simulink model "Resp18e_updatedPulse"  (Simulink 7.3)
settings: Solver=ode23  StartTime=0.0  StopTime=20  FixedStep=0.01  MaxStep=0.05  RelTol=1e-6
values from neighbouring files (symbols this model uses):
  alpha_CO2_brain = 2.9/1e3*760/P_stp/K_stp    (= 0.00097047576489)    [initialize_parameters.m]
  alpha_CO2_fat = 0.9/K_stp/P_stp    (= 0.000396292281489)    [initialize_parameters.m]
  alpha_CO2_heart = 2.4/1e3*760/P_stp/K_stp    (= 0.00080315235715)    [initialize_parameters.m]
  alpha_CO2_lean = 4.2/1e3*760/P_stp/K_stp    (= 0.00140551662501)    [initialize_parameters.m]
  alpha_CO2_lungtiss_fast = alpha_CO2_lungtiss_fast./0.1333    [initialize_parameters.m]
  alpha_CO2_muscle = 4.2/1e3*760/P_stp/K_stp    (= 0.00140551662501)    [initialize_parameters.m]
  alpha_CO2_other = 3.0/1e3*760/P_stp/K_stp    (= 0.00100394044644)    [initialize_parameters.m]
  alpha_O2_fat = 5*0.024/K_stp/P_stp    (= 5.28389708651e-05)    [initialize_parameters.m]
  alpha_O2_tissue = 0.024/K_stp/P_stp    (= 1.0567794173e-05)    [initialize_parameters.m]
  BOHRF0 = O2_SHIFT - T_BLOOD_M_37 * (0.024 + BOHRF * 0.0147) - BOHRF1 * 7.4    (= -3.552)    [initialize_parameters.m]
  BOHRF1 = BOHRF * (1 - T_BLOOD_M_37 * 0.0065)    (= 0.48)    [initialize_parameters.m]
  C_a_CO2_i = 20.8e-3    (= 0.0208)    [initialize_parameters.m]    (also in resp18e_ic_norm.mat = 0.0202734801806)
  C_a_O2_i = 8.95e-3    (= 0.00895)    [initialize_parameters.m]    (also in resp18e_ic_norm.mat = 0.00918087581167)
  CAP_O2 = 0.01 * CAP_O2    (= 0.201)    [initialize_parameters.m]
  Cardiac_duty_cycle = 40    [initialize_parameters.m]
  Co_CO2_brain = 401*K_Co_CO2/1e3/K_stp    (= 0.0107345869894)    [initialize_parameters.m]
  Co_CO2_heart = 487*K_Co_CO2/1e3/K_stp    (= 0.0130367677403)    [initialize_parameters.m]
  Co_CO2_lean = 342*K_Co_CO2/1e3/K_stp    (= 0.00915518391618)    [initialize_parameters.m]
  Co_CO2_muscle = 342*K_Co_CO2/1e3/K_stp    (= 0.00915518391618)    [initialize_parameters.m]
  Co_CO2_other = 355*K_Co_CO2/1e3/K_stp    (= 0.00950318798317)    [initialize_parameters.m]
  DH2ODS = DH2ODS + 0.007 * HB_MEQ * (HB_MEQ - 9) / (13.5 * (13.5 - 9))    (= 0.00498709726946)    [initialize_parameters.m]
  F_insp_alv_alvds = F_v_alv_deadspace / F_insp_hivq    (= 0.00299401197605)    [initialize_parameters.m]
  F_insp_alv_hivq = F_v_alv_hivq      / F_insp_hivq    (= 0.997005988024)    [initialize_parameters.m]
  F_insp_alv_lovq = F_v_alv_lovq      / F_insp_lovq    (= 0.5)    [initialize_parameters.m]
  F_insp_alv_midvq = F_v_alv_midvq     / F_insp_lovq    (= 0.5)    [initialize_parameters.m]
  F_insp_hivq = F_v_alv_deadspace + F_v_alv_hivq    (= 0.334)    [initialize_parameters.m]
  F_insp_lovq = F_v_alv_midvq     + F_v_alv_lovq    (= 0.666)    [initialize_parameters.m]
  Fi_CO2_param_est = 0.01    [initialize_parameters.m]
  Fi_error = 1e-6    (= 1e-06)    [initialize_parameters.m]
  Fi_N2_mean = 1-(Fi_O2_mean + Fi_N2O_mean)    (= 0.65)    [initialize_parameters.m]
  Fi_O2_mean = 0.35    [initialize_parameters.m]
  Fi_O2_param_est = 0.01    [initialize_parameters.m]
  Fq_brain = 0.114    [initialize_parameters.m]
  Fq_error = 1e-8    (= 1e-08)    [initialize_parameters.m]
  Fq_fat = 0.103    [initialize_parameters.m]
  Fq_heart = 0.041    [initialize_parameters.m]
  Fq_hepatic = 0.069    [initialize_parameters.m]
  Fq_kidneys = 0.215    [initialize_parameters.m]
  Fq_lean = 0.090    (= 0.09)    [initialize_parameters.m]
  Fq_lungs_anatomicalshunt = 0.01    [initialize_parameters.m]
  Fq_lungs_hivq = (1-Fq_lungs_pulmshunt-Fq_lungs_anatomicalshunt)    *F_v_alv_hivq/(F_v_alv_hivq+F_v_alv_midvq+F_v_alv_lovq)    (= 0.3)    [initialize_parameters.m]
  Fq_lungs_lovq = (1-Fq_lungs_pulmshunt-Fq_lungs_anatomicalshunt)    *F_v_alv_lovq/(F_v_alv_hivq+F_v_alv_midvq+F_v_alv_lovq)    (= 0.3)    [initialize_parameters.m]
  Fq_lungs_midvq = (1-Fq_lungs_pulmshunt-Fq_lungs_anatomicalshunt)    *F_v_alv_midvq/(F_v_alv_hivq+F_v_alv_midvq+F_v_alv_lovq)    (= 0.3)    [initialize_parameters.m]
  Fq_lungs_pulmshunt = 0.09    [initialize_parameters.m]
  Fq_muscle = 0.096    [initialize_parameters.m]
  Fq_pershunt = 0.101    [initialize_parameters.m]
  Fq_portal = 0.171    [initialize_parameters.m]
  FRC = 2.2    [initialize_parameters.m]
  H2OB = H2OVC + 0.938 * (1 - VC_74)    (= 0.840191964286)    [initialize_parameters.m]
  k_CO2_lungtiss_fast_alvds = k_CO2_lungtiss_fast*F_v_alv_deadspace    (= 3.63090772693e-07)    [initialize_parameters.m]
  k_CO2_lungtiss_fast_hivq = k_CO2_lungtiss_fast*F_v_alv_hivq    (= 0.000120909227307)    [initialize_parameters.m]
  k_CO2_lungtiss_fast_lovq = k_CO2_lungtiss_fast*F_v_alv_lovq    (= 0.000120909227307)    [initialize_parameters.m]
  k_CO2_lungtiss_fast_midvq = k_CO2_lungtiss_fast*F_v_alv_midvq    (= 0.000120909227307)    [initialize_parameters.m]
  k_CO2_lungtiss_slow_alvds = k_CO2_lungtiss_slow*F_v_alv_deadspace    (= 4.95123780945e-09)    [initialize_parameters.m]
  k_CO2_lungtiss_slow_hivq = k_CO2_lungtiss_slow*F_v_alv_hivq    (= 1.64876219055e-06)    [initialize_parameters.m]
  k_CO2_lungtiss_slow_lovq = k_CO2_lungtiss_slow*F_v_alv_lovq    (= 1.64876219055e-06)    [initialize_parameters.m]
  k_CO2_lungtiss_slow_midvq = k_CO2_lungtiss_slow*F_v_alv_midvq    (= 1.64876219055e-06)    [initialize_parameters.m]
  K_diff_CO2_hivq = K_diff_CO2*F_v_alv_hivq    (= 0.0014985)    [initialize_parameters.m]
  K_diff_CO2_lovq = K_diff_CO2*F_v_alv_lovq    (= 0.0014985)    [initialize_parameters.m]
  K_diff_CO2_midvq = K_diff_CO2*F_v_alv_midvq    (= 0.0014985)    [initialize_parameters.m]
  K_diff_O2_hivq = K_diff_O2*F_v_alv_hivq    (= 7.326e-05)    [initialize_parameters.m]
  K_diff_O2_lovq = K_diff_O2*F_v_alv_lovq    (= 7.326e-05)    [initialize_parameters.m]
  K_diff_O2_midvq = K_diff_O2*F_v_alv_midvq    (= 7.326e-05)    [initialize_parameters.m]
  K_exp_alv_alvds = 1/1    (= 1)    [initialize_parameters.m]
  K_exp_alv_hivq = 1/1    (= 1)    [initialize_parameters.m]
  K_press = 760/101.325    (= 7.50061682704)    [initialize_parameters.m]
  K_stp = R*(T_stp+273.15)/(P_stp*1000)    (= 22.4135311621)    [initialize_parameters.m]
  Kg_alv = R*(T_alv+273.15)/(P_baro*1000)    (= 25.3668469802)    [initialize_parameters.m]
  LN10 = 2.30258509299405    (= 2.30258509299)    [initialize_parameters.m]
  m_alv_alvds_i = (FRC-V_deadspace_total)/Kg_alv * F_v_alv_deadspace    [initialize_parameters.m]
  m_alv_hivq_i = (FRC-V_deadspace_total)/Kg_alv * F_v_alv_hivq    [initialize_parameters.m]
  m_alv_lovq_i = (FRC-V_deadspace_total)/Kg_alv * F_v_alv_lovq    [initialize_parameters.m]
  m_alv_midvq_i = (FRC-V_deadspace_total)/Kg_alv * F_v_alv_midvq    [initialize_parameters.m]
  m_CO2_alv_alvds_i = F_CO2_i * m_alv_alvds_i    [initialize_parameters.m]
  m_CO2_alv_hivq_i = F_CO2_i * m_alv_hivq_i    [initialize_parameters.m]
  m_CO2_alv_lovq_i = F_CO2_i * m_alv_lovq_i    [initialize_parameters.m]
  m_CO2_alv_midvq_i = F_CO2_i * m_alv_midvq_i    [initialize_parameters.m]
  m_CO2_brain_b_i = C_a_CO2_i*Vb_brain    (= 0.002184)    [initialize_parameters.m]
  m_CO2_brain_t_i = (Co_CO2_brain  + alpha_CO2_brain *P_v_CO2_i)* Vt_brain    (= 0.0171268217946)    [initialize_parameters.m]
  m_CO2_common_b_i = C_a_CO2_i*Vb_common    (= 0.0170421333333)    [initialize_parameters.m]
  m_CO2_ds0_i = F_CO2_i*m_ds0_i    (= 0.000985538329597)    [initialize_parameters.m]
  m_CO2_ds_large_i = F_CO2_i * m_deadspace_large_1    [initialize_parameters.m]
  m_CO2_ds_med_hivq1_i = F_CO2_i * m_deadspace_med_hivq_1    [initialize_parameters.m]
  m_CO2_ds_med_hivq2_i = F_CO2_i * m_deadspace_med_hivq_2    [initialize_parameters.m]
  m_CO2_ds_med_lovq1_i = F_CO2_i * m_deadspace_med_lovq_1    [initialize_parameters.m]
  m_CO2_ds_med_lovq2_i = F_CO2_i * m_deadspace_med_lovq_2    [initialize_parameters.m]
  m_CO2_ds_small_alvds_i = F_CO2_i * m_deadspace_small_alvdeadspace    [initialize_parameters.m]
  m_CO2_ds_small_hivq_i = F_CO2_i * m_deadspace_small_hivq    [initialize_parameters.m]
  m_CO2_ds_small_lovq_i = F_CO2_i * m_deadspace_small_lovq    [initialize_parameters.m]
  m_CO2_ds_small_midvq_i = F_CO2_i * m_deadspace_small_midvq    [initialize_parameters.m]
  m_CO2_fat_b_i = C_a_CO2_i*Vb_fat    (= 0.0116896)    [initialize_parameters.m]
  m_CO2_fat_t_i = P_a_CO2_i*alpha_CO2_fat*Vt_fat    (= 0.0302752719501)    [initialize_parameters.m]
  m_CO2_heart_b_i = C_a_CO2_i*Vb_heart    (= 0.000832)    [initialize_parameters.m]
  m_CO2_heart_t_i = (Co_CO2_heart  + alpha_CO2_heart *P_v_CO2_i)* Vt_heart    (= 0.00402544335149)    [initialize_parameters.m]
  m_CO2_hepatic_b_i = C_a_CO2_i*Vb_hepatic    (= 0.0019136)    [initialize_parameters.m]
  m_CO2_kidneys_b_i = C_a_CO2_i*Vb_kidneys    (= 0.0012064)    [initialize_parameters.m]
  m_CO2_kidneys_t_i = (Co_CO2_other  + alpha_CO2_other *P_v_CO2_i)* Vt_kidneys    (= 0.0045902552907)    [initialize_parameters.m]
  m_CO2_lean_b_i = C_a_CO2_i*Vb_lean    (= 0.0191984)    [initialize_parameters.m]
  m_CO2_lean_t_i = (Co_CO2_lean   + alpha_CO2_lean  *P_v_CO2_i)* Vt_lean    (= 0.0884995401953)    [initialize_parameters.m]
  m_CO2_liver_t_i = (Co_CO2_other  + alpha_CO2_other *P_v_CO2_i)* Vt_liver    (= 0.0187019339777)    [initialize_parameters.m]
  m_CO2_lungtiss_fast_alvds_i = F_CO2_i*(P_baro-P_A_H2O)*V_lungtiss_alvds *alpha_CO2_lungtiss_fast(2)    [initialize_parameters.m]
  m_CO2_lungtiss_fast_hivq_i = F_CO2_i*(P_baro-P_A_H2O)*V_lungtiss_hivq  *alpha_CO2_lungtiss_fast(2)    [initialize_parameters.m]
  m_CO2_lungtiss_fast_lovq_i = F_CO2_i*(P_baro-P_A_H2O)*V_lungtiss_lovq  *alpha_CO2_lungtiss_fast(2)    [initialize_parameters.m]
  m_CO2_lungtiss_fast_midvq_i = F_CO2_i*(P_baro-P_A_H2O)*V_lungtiss_midvq *alpha_CO2_lungtiss_fast(2)    [initialize_parameters.m]
  m_CO2_lungtiss_slow_alvds_i = F_CO2_i*(P_baro-P_A_H2O)*V_lungtiss_alvds*alpha_CO2_lungtiss_slow    [initialize_parameters.m]
  m_CO2_lungtiss_slow_hivq_i = F_CO2_i*(P_baro-P_A_H2O)*V_lungtiss_hivq *alpha_CO2_lungtiss_slow    [initialize_parameters.m]
  m_CO2_lungtiss_slow_lovq_i = F_CO2_i*(P_baro-P_A_H2O)*V_lungtiss_lovq *alpha_CO2_lungtiss_slow    [initialize_parameters.m]
  m_CO2_lungtiss_slow_midvq_i = F_CO2_i*(P_baro-P_A_H2O)*V_lungtiss_midvq*alpha_CO2_lungtiss_slow    [initialize_parameters.m]
  m_CO2_LV_b_i = C_a_CO2_i*Vb_LV    (= 0.00391733333333)    [initialize_parameters.m]
  m_CO2_muscle_b_i = C_a_CO2_i*Vb_muscle    (= 0.0201344)    [initialize_parameters.m]
  m_CO2_muscle_t_i = (Co_CO2_muscle + alpha_CO2_muscle*P_v_CO2_i)* Vt_muscle    (= 0.363660431061)    [initialize_parameters.m]
  m_CO2_pershunt_b_i = C_a_CO2_i*Vb_pershunt    (= 0.0027248)    [initialize_parameters.m]
  m_CO2_portal_b_i = C_a_CO2_i*Vb_portal    (= 0.0210912)    [initialize_parameters.m]
  m_CO2_portal_t_i = (Co_CO2_other  + alpha_CO2_other *P_v_CO2_i)* Vt_portal    (= 0.0164739329706)    [initialize_parameters.m]
  m_CO2_pulmcap_b_hivq_i = C_a_CO2_i*Vb_pulmcap_hivq    (= 0.000630933333333)    [initialize_parameters.m]
  m_CO2_pulmcap_b_lovq_i = C_a_CO2_i*Vb_pulmcap_lovq    (= 0.000630933333333)    [initialize_parameters.m]
  m_CO2_pulmcap_b_midvq_i = C_a_CO2_i*Vb_pulmcap_midvq    (= 0.000630933333333)    [initialize_parameters.m]
  m_CO2_pulmcap_b_pulmshunt_i = C_a_CO2_i*Vb_pulmcap_pulmshunt    (= 0.0001872)    [initialize_parameters.m]
  m_CO2_RV_b_i = C_v_CO2_i*Vb_RV    (= 0.004181)    [initialize_parameters.m]
  m_N2_alv_alvds_i = Fi_N2_mean * (m_alv_alvds_i - m_CO2_alv_alvds_i)    [initialize_parameters.m]
  ... (+122 more)
undefined symbols (not defined in the file or in its folder): AH2OVC, AHCO3B, DHCO3BDS, litres, mole
libraries: simulink x28
(part 7 of 8)

== system Resp18e_updatedPulse/Patient/Kidneys/Kidneys/Blood gas curves Olszowka SI Units ==
  P_CO2 : Inport  OutDataType=sfix(16)  OutScaling=2^0
  P_O2 : Inport  Port=2  OutDataType=sfix(16)  OutScaling=2^0
  Olszowka's diss curves : Subsystem
  kPa > mm Hg : Gain  Gain=K_press  ParameterDataType=sfix(16)  ParameterScaling=2^0  OutDataType=sfix(16)  OutScaling=2^0  SaturateOnIntegerOverflow=on  OutDataTypeStr=Inherit: Same as input  ParamDataTypeStr=Inherit: Same as input
  kPa > mm Hg1 : Gain  Gain=K_press  ParameterDataType=sfix(16)  ParameterScaling=2^0  OutDataType=sfix(16)  OutScaling=2^0  SaturateOnIntegerOverflow=on  OutDataTypeStr=Inherit: Same as input  ParamDataTypeStr=Inherit: Same as input
  l > mole : Gain  Gain=1/K_stp  ParameterDataType=sfix(16)  ParameterScaling=2^0  OutDataType=sfix(16)  OutScaling=2^0  SaturateOnIntegerOverflow=on  OutDataTypeStr=Inherit: Same as input  ParamDataTypeStr=Inherit: Same as input
  l> mole : Gain  Gain=1/K_stp  ParameterDataType=sfix(16)  ParameterScaling=2^0  OutDataType=sfix(16)  OutScaling=2^0  SaturateOnIntegerOverflow=on  OutDataTypeStr=Inherit: Same as input  ParamDataTypeStr=Inherit: Same as input
  C_CO2 : Outport  OutDataType=sfix(16)  OutScaling=2^0
  C_O2 : Outport  Port=2  OutDataType=sfix(16)  OutScaling=2^0
  wires:
  kPa > mm Hg/1 -> Olszowka's diss curves/1(P_CO2)
  kPa > mm Hg1/1 -> Olszowka's diss curves/2(PO2)
  Olszowka's diss curves/1(C_CO2) -> l > mole/1
  Olszowka's diss curves/2(C_O2) -> l> mole/1
  l > mole/1 -> C_CO2/1
  P_CO2/1 -> kPa > mm Hg/1
  l> mole/1 -> C_O2/1
  P_O2/1 -> kPa > mm Hg1/1

== system Resp18e_updatedPulse/Patient/Kidneys/Kidneys/InvTissue diss curves ==
  note: kPa
  note: mole/l
  C_CO2 : Inport  OutDataType=sfix(16)  OutScaling=2^0
  C_O2 : Inport  Port=2  OutDataType=sfix(16)  OutScaling=2^0
  " " : Fcn  Expr=u(1)/alpha_O2_tissue
  q1 : Fcn  Expr=(u(1)-Co_CO2_other)/alpha_CO2_other
  P_CO2 : Outport  OutDataType=sfix(16)  OutScaling=2^0
  P_O2 : Outport  Port=2  OutDataType=sfix(16)  OutScaling=2^0
  wires:
  " "/1 -> P_O2/1  "PTO2"
  C_O2/1 -> " "/1
  C_CO2/1 -> q1/1
  q1/1 -> P_CO2/1  "PCO2"

== system Resp18e_updatedPulse/Patient/LV + Aorta/Arterial blood gas measurements/Olszowka SI units ==
  C_CO2 : Inport  OutDataType=sfix(16)  OutScaling=2^0
  C_O2 : Inport  Port=2  OutDataType=sfix(16)  OutScaling=2^0
  Olszowka's diss curves : Subsystem
  mmHg>kPa : Gain  Gain=1/K_press  ParameterDataType=sfix(16)  ParameterScaling=2^0  OutDataType=sfix(16)  OutScaling=2^0  SaturateOnIntegerOverflow=on  OutDataTypeStr=Inherit: Same as input  ParamDataTypeStr=Inherit: Same as input
  mmHg>kPa1 : Gain  Gain=1/K_press  ParameterDataType=sfix(16)  ParameterScaling=2^0  OutDataType=sfix(16)  OutScaling=2^0  SaturateOnIntegerOverflow=on  OutDataTypeStr=Inherit: Same as input  ParamDataTypeStr=Inherit: Same as input
  mole > l : Gain  Gain=K_stp  ParameterDataType=sfix(16)  ParameterScaling=2^0  OutDataType=sfix(16)  OutScaling=2^0  SaturateOnIntegerOverflow=on  OutDataTypeStr=Inherit: Same as input  ParamDataTypeStr=Inherit: Same as input
  mole>l : Gain  Gain=K_stp  ParameterDataType=sfix(16)  ParameterScaling=2^0  OutDataType=sfix(16)  OutScaling=2^0  SaturateOnIntegerOverflow=on  OutDataTypeStr=Inherit: Same as input  ParamDataTypeStr=Inherit: Same as input
  P_CO2 : Outport  OutDataType=sfix(16)  OutScaling=2^0
  P_O2 : Outport  Port=2  OutDataType=sfix(16)  OutScaling=2^0
  pH : Outport  Port=3  OutDataType=sfix(16)  OutScaling=2^0
  Sat : Outport  Port=4  OutDataType=sfix(16)  OutScaling=2^0
  wires:
  C_CO2/1 -> mole>l/1
  mole>l/1 -> Olszowka's diss curves/1(C_CO2)
  mole > l/1 -> Olszowka's diss curves/2(C_O2)
  Olszowka's diss curves/1(P_CO2) -> mmHg>kPa1/1
  Olszowka's diss curves/2(P_O2) -> mmHg>kPa/1
  mmHg>kPa1/1 -> P_CO2/1
  mmHg>kPa/1 -> P_O2/1
  Olszowka's diss curves/3(pH) -> pH/1
  C_O2/1 -> mole > l/1
  Olszowka's diss curves/4(Sat) -> Sat/1

== system Resp18e_updatedPulse/Patient/Large Veins/Mixed venous measurements/Olszowka SI units ==
  C_CO2 : Inport  OutDataType=sfix(16)  OutScaling=2^0
  C_O2 : Inport  Port=2  OutDataType=sfix(16)  OutScaling=2^0
  Olszowka's diss curves : Subsystem
  mmHg>kPa : Gain  Gain=1/K_press  ParameterDataType=sfix(16)  ParameterScaling=2^0  OutDataType=sfix(16)  OutScaling=2^0  SaturateOnIntegerOverflow=on  OutDataTypeStr=Inherit: Same as input  ParamDataTypeStr=Inherit: Same as input
  mmHg>kPa1 : Gain  Gain=1/K_press  ParameterDataType=sfix(16)  ParameterScaling=2^0  OutDataType=sfix(16)  OutScaling=2^0  SaturateOnIntegerOverflow=on  OutDataTypeStr=Inherit: Same as input  ParamDataTypeStr=Inherit: Same as input
  mole > l : Gain  Gain=K_stp  ParameterDataType=sfix(16)  ParameterScaling=2^0  OutDataType=sfix(16)  OutScaling=2^0  SaturateOnIntegerOverflow=on  OutDataTypeStr=Inherit: Same as input  ParamDataTypeStr=Inherit: Same as input
  mole>l : Gain  Gain=K_stp  ParameterDataType=sfix(16)  ParameterScaling=2^0  OutDataType=sfix(16)  OutScaling=2^0  SaturateOnIntegerOverflow=on  OutDataTypeStr=Inherit: Same as input  ParamDataTypeStr=Inherit: Same as input
  P_CO2 : Outport  OutDataType=sfix(16)  OutScaling=2^0
  P_O2 : Outport  Port=2  OutDataType=sfix(16)  OutScaling=2^0
  pH : Outport  Port=3  OutDataType=sfix(16)  OutScaling=2^0
  wires:
  Olszowka's diss curves/3(pH) -> pH/1
  mmHg>kPa/1 -> P_O2/1
  mmHg>kPa1/1 -> P_CO2/1
  Olszowka's diss curves/2(P_O2) -> mmHg>kPa/1
  Olszowka's diss curves/1(P_CO2) -> mmHg>kPa1/1
  mole > l/1 -> Olszowka's diss curves/2(C_O2)
  C_O2/1 -> mole > l/1
  mole>l/1 -> Olszowka's diss curves/1(C_CO2)
  C_CO2/1 -> mole>l/1

== system Resp18e_updatedPulse/Patient/Liver & gut/Liver/Blood gas curves Olszowka SI Units ==
  P_CO2 : Inport  OutDataType=sfix(16)  OutScaling=2^0
  P_O2 : Inport  Port=2  OutDataType=sfix(16)  OutScaling=2^0
  Olszowka's diss curves : Subsystem
  kPa > mm Hg : Gain  Gain=K_press  ParameterDataType=sfix(16)  ParameterScaling=2^0  OutDataType=sfix(16)  OutScaling=2^0  SaturateOnIntegerOverflow=on  OutDataTypeStr=Inherit: Same as input  ParamDataTypeStr=Inherit: Same as input
  kPa > mm Hg1 : Gain  Gain=K_press  ParameterDataType=sfix(16)  ParameterScaling=2^0  OutDataType=sfix(16)  OutScaling=2^0  SaturateOnIntegerOverflow=on  OutDataTypeStr=Inherit: Same as input  ParamDataTypeStr=Inherit: Same as input
  l > mole : Gain  Gain=1/K_stp  ParameterDataType=sfix(16)  ParameterScaling=2^0  OutDataType=sfix(16)  OutScaling=2^0  SaturateOnIntegerOverflow=on  OutDataTypeStr=Inherit: Same as input  ParamDataTypeStr=Inherit: Same as input
  l> mole : Gain  Gain=1/K_stp  ParameterDataType=sfix(16)  ParameterScaling=2^0  OutDataType=sfix(16)  OutScaling=2^0  SaturateOnIntegerOverflow=on  OutDataTypeStr=Inherit: Same as input  ParamDataTypeStr=Inherit: Same as input
  C_CO2 : Outport  OutDataType=sfix(16)  OutScaling=2^0
  C_O2 : Outport  Port=2  OutDataType=sfix(16)  OutScaling=2^0
  wires:
  kPa > mm Hg/1 -> Olszowka's diss curves/1(P_CO2)
  kPa > mm Hg1/1 -> Olszowka's diss curves/2(PO2)
  Olszowka's diss curves/1(C_CO2) -> l > mole/1
  Olszowka's diss curves/2(C_O2) -> l> mole/1
  l > mole/1 -> C_CO2/1
  P_CO2/1 -> kPa > mm Hg/1
  l> mole/1 -> C_O2/1
  P_O2/1 -> kPa > mm Hg1/1

== system Resp18e_updatedPulse/Patient/Liver & gut/Liver/InvTissue diss curves ==
  note: mole/l
  note: kPa
  C_CO2 : Inport  OutDataType=sfix(16)  OutScaling=2^0
  C_O2 : Inport  Port=2  OutDataType=sfix(16)  OutScaling=2^0
  " " : Fcn  Expr=u(1)/alpha_O2_tissue
  q1 : Fcn  Expr=(u(1)-Co_CO2_other)/alpha_CO2_other
  P_CO2 : Outport  OutDataType=sfix(16)  OutScaling=2^0
  P_O2 : Outport  Port=2  OutDataType=sfix(16)  OutScaling=2^0
  wires:
  C_O2/1 -> " "/1
  " "/1 -> P_O2/1  "PTO2"
  C_CO2/1 -> q1/1
  q1/1 -> P_CO2/1  "PCO2"

== system Resp18e_updatedPulse/Patient/Liver & gut/Portal/Blood gas curves Olszowka SI Units ==
  P_CO2 : Inport  OutDataType=sfix(16)  OutScaling=2^0
  P_O2 : Inport  Port=2  OutDataType=sfix(16)  OutScaling=2^0
  Olszowka's diss curves : Subsystem
  kPa > mm Hg : Gain  Gain=K_press  ParameterDataType=sfix(16)  ParameterScaling=2^0  OutDataType=sfix(16)  OutScaling=2^0  SaturateOnIntegerOverflow=on  OutDataTypeStr=Inherit: Same as input  ParamDataTypeStr=Inherit: Same as input
  kPa > mm Hg1 : Gain  Gain=K_press  ParameterDataType=sfix(16)  ParameterScaling=2^0  OutDataType=sfix(16)  OutScaling=2^0  SaturateOnIntegerOverflow=on  OutDataTypeStr=Inherit: Same as input  ParamDataTypeStr=Inherit: Same as input
  l > mole : Gain  Gain=1/K_stp  ParameterDataType=sfix(16)  ParameterScaling=2^0  OutDataType=sfix(16)  OutScaling=2^0  SaturateOnIntegerOverflow=on  OutDataTypeStr=Inherit: Same as input  ParamDataTypeStr=Inherit: Same as input
  l> mole : Gain  Gain=1/K_stp  ParameterDataType=sfix(16)  ParameterScaling=2^0  OutDataType=sfix(16)  OutScaling=2^0  SaturateOnIntegerOverflow=on  OutDataTypeStr=Inherit: Same as input  ParamDataTypeStr=Inherit: Same as input
  C_CO2 : Outport  OutDataType=sfix(16)  OutScaling=2^0
  C_O2 : Outport  Port=2  OutDataType=sfix(16)  OutScaling=2^0
  wires:
  kPa > mm Hg/1 -> Olszowka's diss curves/1(P_CO2)
  kPa > mm Hg1/1 -> Olszowka's diss curves/2(PO2)
  Olszowka's diss curves/1(C_CO2) -> l > mole/1
  Olszowka's diss curves/2(C_O2) -> l> mole/1
  l > mole/1 -> C_CO2/1
  P_CO2/1 -> kPa > mm Hg/1
  l> mole/1 -> C_O2/1
  P_O2/1 -> kPa > mm Hg1/1

== system Resp18e_updatedPulse/Patient/Liver & gut/Portal/InvTissue diss curves ==
  note: kPa
  note: mole/l
  note: mole/l
  C_CO2 : Inport  OutDataType=sfix(16)  OutScaling=2^0
  C_O2 : Inport  Port=2  OutDataType=sfix(16)  OutScaling=2^0
  " " : Fcn  Expr=u(1)/alpha_O2_tissue
  q1 : Fcn  Expr=(u(1)-Co_CO2_other)/alpha_CO2_other
  P_CO2 : Outport  OutDataType=sfix(16)  OutScaling=2^0
  PT_O2 : Outport  Port=2  OutDataType=sfix(16)  OutScaling=2^0
  wires:
  " "/1 -> PT_O2/1  "PO2"
  C_O2/1 -> " "/1
  C_CO2/1 -> q1/1
  q1/1 -> P_CO2/1  "PCO2"

== system Resp18e_updatedPulse/Patient/Muscle/Muscle/Blood gas curves Olszowka SI Units ==
  P_CO2 : Inport  OutDataType=sfix(16)  OutScaling=2^0
  P_O2 : Inport  Port=2  OutDataType=sfix(16)  OutScaling=2^0
  Olszowka's diss curves : Subsystem
  kPa > mm Hg : Gain  Gain=K_press  ParameterDataType=sfix(16)  ParameterScaling=2^0  OutDataType=sfix(16)  OutScaling=2^0  SaturateOnIntegerOverflow=on  OutDataTypeStr=Inherit: Same as input  ParamDataTypeStr=Inherit: Same as input
  kPa > mm Hg1 : Gain  Gain=K_press  ParameterDataType=sfix(16)  ParameterScaling=2^0  OutDataType=sfix(16)  OutScaling=2^0  SaturateOnIntegerOverflow=on  OutDataTypeStr=Inherit: Same as input  ParamDataTypeStr=Inherit: Same as input
  l > mole : Gain  Gain=1/K_stp  ParameterDataType=sfix(16)  ParameterScaling=2^0  OutDataType=sfix(16)  OutScaling=2^0  SaturateOnIntegerOverflow=on  OutDataTypeStr=Inherit: Same as input  ParamDataTypeStr=Inherit: Same as input
  l> mole : Gain  Gain=1/K_stp  ParameterDataType=sfix(16)  ParameterScaling=2^0  OutDataType=sfix(16)  OutScaling=2^0  SaturateOnIntegerOverflow=on  OutDataTypeStr=Inherit: Same as input  ParamDataTypeStr=Inherit: Same as input
  C_CO2 : Outport  OutDataType=sfix(16)  OutScaling=2^0
  C_O2 : Outport  Port=2  OutDataType=sfix(16)  OutScaling=2^0
  wires:
  kPa > mm Hg/1 -> Olszowka's diss curves/1(P_CO2)
  kPa > mm Hg1/1 -> Olszowka's diss curves/2(PO2)
  Olszowka's diss curves/1(C_CO2) -> l > mole/1
  Olszowka's diss curves/2(C_O2) -> l> mole/1
  l > mole/1 -> C_CO2/1
  P_CO2/1 -> kPa > mm Hg/1
  l> mole/1 -> C_O2/1
  P_O2/1 -> kPa > mm Hg1/1

== system Resp18e_updatedPulse/Patient/Muscle/Muscle/InvTissue diss curves ==
  note: mole/l
  note: kPa
  C_CO2 : Inport  OutDataType=sfix(16)  OutScaling=2^0
  C_O2 : Inport  Port=2  OutDataType=sfix(16)  OutScaling=2^0
  " " : Fcn  Expr=u(1)/alpha_O2_tissue
  q1 : Fcn  Expr=(u(1)-Co_CO2_muscle)/alpha_CO2_muscle
  P_CO2 : Outport  OutDataType=sfix(16)  OutScaling=2^0
  P_O2 : Outport  Port=2  OutDataType=sfix(16)  OutScaling=2^0
  wires:
  C_CO2/1 -> q1/1
  q1/1 -> P_CO2/1  "PCO2"
  C_O2/1 -> " "/1
  " "/1 -> P_O2/1  "PO2"

== system Resp18e_updatedPulse/Patient/Other lean/Lean/Blood gas curves Olszowka SI Units ==
  P_CO2 : Inport  OutDataType=sfix(16)  OutScaling=2^0
  P_O2 : Inport  Port=2  OutDataType=sfix(16)  OutScaling=2^0
  Olszowka's diss curves : Subsystem
  kPa > mm Hg : Gain  Gain=K_press  ParameterDataType=sfix(16)  ParameterScaling=2^0  OutDataType=sfix(16)  OutScaling=2^0  SaturateOnIntegerOverflow=on  OutDataTypeStr=Inherit: Same as input  ParamDataTypeStr=Inherit: Same as input
  kPa > mm Hg1 : Gain  Gain=K_press  ParameterDataType=sfix(16)  ParameterScaling=2^0  OutDataType=sfix(16)  OutScaling=2^0  SaturateOnIntegerOverflow=on  OutDataTypeStr=Inherit: Same as input  ParamDataTypeStr=Inherit: Same as input
  l > mole : Gain  Gain=1/K_stp  ParameterDataType=sfix(16)  ParameterScaling=2^0  OutDataType=sfix(16)  OutScaling=2^0  SaturateOnIntegerOverflow=on  OutDataTypeStr=Inherit: Same as input  ParamDataTypeStr=Inherit: Same as input
  l> mole : Gain  Gain=1/K_stp  ParameterDataType=sfix(16)  ParameterScaling=2^0  OutDataType=sfix(16)  OutScaling=2^0  SaturateOnIntegerOverflow=on  OutDataTypeStr=Inherit: Same as input  ParamDataTypeStr=Inherit: Same as input
  C_CO2 : Outport  OutDataType=sfix(16)  OutScaling=2^0
  C_O2 : Outport  Port=2  OutDataType=sfix(16)  OutScaling=2^0
  wires:
  kPa > mm Hg/1 -> Olszowka's diss curves/1(P_CO2)
  kPa > mm Hg1/1 -> Olszowka's diss curves/2(PO2)
  Olszowka's diss curves/1(C_CO2) -> l > mole/1
  Olszowka's diss curves/2(C_O2) -> l> mole/1
  l > mole/1 -> C_CO2/1
  P_CO2/1 -> kPa > mm Hg/1
  l> mole/1 -> C_O2/1
  P_O2/1 -> kPa > mm Hg1/1

== system Resp18e_updatedPulse/Patient/Other lean/Lean/InvTissue diss curves ==
  note: kPa
  note: mole/l
  note: Use same dissociation constants as muscle compartment
      | because protein content is high (see Mapleson #193)
  C_CO2 : Inport  OutDataType=sfix(16)  OutScaling=2^0
  C_O2 : Inport  Port=2  OutDataType=sfix(16)  OutScaling=2^0
  " " : Fcn  Expr=u(1)/alpha_O2_tissue
  q1 : Fcn  Expr=(u(1)-Co_CO2_lean)/alpha_CO2_lean
  P_CO2 : Outport  OutDataType=sfix(16)  OutScaling=2^0
  P_O2 : Outport  Port=2  OutDataType=sfix(16)  OutScaling=2^0
  wires:
  " "/1 -> P_O2/1  "PO2"
  C_O2/1 -> " "/1
  C_CO2/1 -> q1/1
  q1/1 -> P_CO2/1  "PCO2"

== system Resp18e_updatedPulse/Patient/Pulm cap Hi V/Q/Pulm capillaries/Olszowka SI units ==
  C_CO2 : Inport  OutDataType=sfix(16)  OutScaling=2^0
  C_O2 : Inport  Port=2  OutDataType=sfix(16)  OutScaling=2^0
  Olszowka's diss curves : Subsystem
  mmHg>kPa : Gain  Gain=1/K_press  ParameterDataType=sfix(16)  ParameterScaling=2^0  OutDataType=sfix(16)  OutScaling=2^0  SaturateOnIntegerOverflow=on  OutDataTypeStr=Inherit: Same as input  ParamDataTypeStr=Inherit: Same as input
  mmHg>kPa1 : Gain  Gain=1/K_press  ParameterDataType=sfix(16)  ParameterScaling=2^0  OutDataType=sfix(16)  OutScaling=2^0  SaturateOnIntegerOverflow=on  OutDataTypeStr=Inherit: Same as input  ParamDataTypeStr=Inherit: Same as input
  mole > l : Gain  Gain=K_stp  ParameterDataType=sfix(16)  ParameterScaling=2^0  OutDataType=sfix(16)  OutScaling=2^0  SaturateOnIntegerOverflow=on  OutDataTypeStr=Inherit: Same as input  ParamDataTypeStr=Inherit: Same as input
  mole>l : Gain  Gain=K_stp  ParameterDataType=sfix(16)  ParameterScaling=2^0  OutDataType=sfix(16)  OutScaling=2^0  SaturateOnIntegerOverflow=on  OutDataTypeStr=Inherit: Same as input  ParamDataTypeStr=Inherit: Same as input
  P_CO2 : Outport  OutDataType=sfix(16)  OutScaling=2^0
  P_O2 : Outport  Port=2  OutDataType=sfix(16)  OutScaling=2^0
  wires:
  mmHg>kPa/1 -> P_O2/1
  Olszowka's diss curves/2(P_O2) -> mmHg>kPa/1
  Olszowka's diss curves/1(P_CO2) -> mmHg>kPa1/1
  mole > l/1 -> Olszowka's diss curves/2(C_O2)
  C_O2/1 -> mole > l/1
  mole>l/1 -> Olszowka's diss curves/1(C_CO2)
  C_CO2/1 -> mole>l/1
  mmHg>kPa1/1 -> P_CO2/1

== system Resp18e_updatedPulse/Patient/Pulm cap Lo V/Q/Pulm capillaries/Olszowka SI units ==
  C_CO2 : Inport  OutDataType=sfix(16)  OutScaling=2^0
  C_O2 : Inport  Port=2  OutDataType=sfix(16)  OutScaling=2^0
  Olszowka's diss curves : Subsystem
  mmHg>kPa : Gain  Gain=1/K_press  ParameterDataType=sfix(16)  ParameterScaling=2^0  OutDataType=sfix(16)  OutScaling=2^0  SaturateOnIntegerOverflow=on  OutDataTypeStr=Inherit: Same as input  ParamDataTypeStr=Inherit: Same as input
  mmHg>kPa1 : Gain  Gain=1/K_press  ParameterDataType=sfix(16)  ParameterScaling=2^0  OutDataType=sfix(16)  OutScaling=2^0  SaturateOnIntegerOverflow=on  OutDataTypeStr=Inherit: Same as input  ParamDataTypeStr=Inherit: Same as input
  mole > l : Gain  Gain=K_stp  ParameterDataType=sfix(16)  ParameterScaling=2^0  OutDataType=sfix(16)  OutScaling=2^0  SaturateOnIntegerOverflow=on  OutDataTypeStr=Inherit: Same as input  ParamDataTypeStr=Inherit: Same as input
  mole>l : Gain  Gain=K_stp  ParameterDataType=sfix(16)  ParameterScaling=2^0  OutDataType=sfix(16)  OutScaling=2^0  SaturateOnIntegerOverflow=on  OutDataTypeStr=Inherit: Same as input  ParamDataTypeStr=Inherit: Same as input
  P_CO2 : Outport  OutDataType=sfix(16)  OutScaling=2^0
  P_O2 : Outport  Port=2  OutDataType=sfix(16)  OutScaling=2^0
  wires:
  mmHg>kPa/1 -> P_O2/1
  Olszowka's diss curves/2(P_O2) -> mmHg>kPa/1
  Olszowka's diss curves/1(P_CO2) -> mmHg>kPa1/1
  mole > l/1 -> Olszowka's diss curves/2(C_O2)
  C_O2/1 -> mole > l/1
  mole>l/1 -> Olszowka's diss curves/1(C_CO2)
  C_CO2/1 -> mole>l/1
  mmHg>kPa1/1 -> P_CO2/1

== system Resp18e_updatedPulse/Patient/Pulm cap Mid V/Q/Pulm capillaries/Olszowka SI units ==
  C_CO2 : Inport  OutDataType=sfix(16)  OutScaling=2^0
  C_O2 : Inport  Port=2  OutDataType=sfix(16)  OutScaling=2^0
  Olszowka's diss curves : Subsystem
  mmHg>kPa : Gain  Gain=1/K_press  ParameterDataType=sfix(16)  ParameterScaling=2^0  OutDataType=sfix(16)  OutScaling=2^0  SaturateOnIntegerOverflow=on  OutDataTypeStr=Inherit: Same as input  ParamDataTypeStr=Inherit: Same as input
  mmHg>kPa1 : Gain  Gain=1/K_press  ParameterDataType=sfix(16)  ParameterScaling=2^0  OutDataType=sfix(16)  OutScaling=2^0  SaturateOnIntegerOverflow=on  OutDataTypeStr=Inherit: Same as input  ParamDataTypeStr=Inherit: Same as input
  mole > l : Gain  Gain=K_stp  ParameterDataType=sfix(16)  ParameterScaling=2^0  OutDataType=sfix(16)  OutScaling=2^0  SaturateOnIntegerOverflow=on  OutDataTypeStr=Inherit: Same as input  ParamDataTypeStr=Inherit: Same as input
  mole>l : Gain  Gain=K_stp  ParameterDataType=sfix(16)  ParameterScaling=2^0  OutDataType=sfix(16)  OutScaling=2^0  SaturateOnIntegerOverflow=on  OutDataTypeStr=Inherit: Same as input  ParamDataTypeStr=Inherit: Same as input
  P_CO2 : Outport  OutDataType=sfix(16)  OutScaling=2^0
  P_O2 : Outport  Port=2  OutDataType=sfix(16)  OutScaling=2^0
  wires:
  mmHg>kPa1/1 -> P_CO2/1
  C_CO2/1 -> mole>l/1
  mole>l/1 -> Olszowka's diss curves/1(C_CO2)
  C_O2/1 -> mole > l/1
  mole > l/1 -> Olszowka's diss curves/2(C_O2)
  Olszowka's diss curves/1(P_CO2) -> mmHg>kPa1/1
  Olszowka's diss curves/2(P_O2) -> mmHg>kPa/1
  mmHg>kPa/1 -> P_O2/1

== system Resp18e_updatedPulse/Patient/Anaesthetic Machine & resp mechanics/Insp gas mixing/Insp gas calcs/CO2 Resp PWM ==
  Compare To Constant : simulink/Logic and Bit Operations/Compare To Constant  SystemSampleTime=-1  relop=>=  const=1.0  LogicOutDataTypeMode=boolean  ZeroCross=off
  Compare To Zero : simulink/Logic and Bit Operations/Compare To Zero  SystemSampleTime=-1  relop=<=  LogicOutDataTypeMode=uint8  ZeroCross=off
  Data Type Conversion : DataTypeConversion  OutDataTypeMode=double  OutDataType=fixdt(1, 16)  OutScaling=2^0  OutDataTypeStr=double
  From Workspace : FromWorkspace  VariableName=mod_duty_cycle  SampleTime=0  Interpolate=off  OutputAfterFinalValue=Holding final value
  From Workspace1 : FromWorkspace  VariableName=mod_resp_rate  SampleTime=0  Interpolate=off  OutputAfterFinalValue=Holding final value
  Integrator : Integrator  ExternalReset=rising  UpperSaturationLimit=1  LowerSaturationLimit=0  ZeroCross=off
  Sub : Sum  Inputs=+-  OutDataType=fixdt(1, 16)  OutScaling=2^-10
  Out1 : Outport  OutDataType=fixdt(1, 16)  OutScaling=2^0
  wires:
  From Workspace/1 -> Sub/2
  Integrator/1 -> Compare To Constant/1, Sub/1
  Sub/1 -> Compare To Zero/1
  Compare To Constant/1 -> Integrator/2
  From Workspace1/1 -> Integrator/1
  Data Type Conversion/1 -> Out1/1
  Compare To Zero/1 -> Data Type Conversion/1

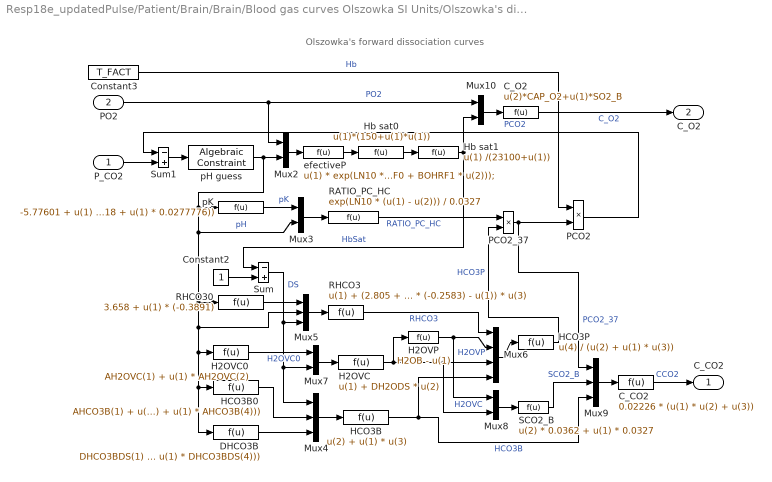
== system Resp18e_updatedPulse/Patient/Brain/Brain/Blood gas curves Olszowka SI Units/Olszowka's diss curves ==
  note: Olszowka's forward dissociation curves
  P_CO2 : Inport  OutDataType=sfix(16)  OutScaling=2^0
  PO2 : Inport  Port=2  OutDataType=sfix(16)  OutScaling=2^0
  "C_CO2 " : Fcn  Expr=0.02226 * (u(1) * u(2) + u(3))
  "C_O2 " : Fcn  Expr=u(2)*CAP_O2+u(1)*SO2_B
  Constant2 : Constant  OutDataType=sfix(16)  OutScaling=2^0
  Constant3 : Constant  Value=T_FACT  OutDataType=sfix(16)  OutScaling=2^0
  DHCO3B : Fcn  Expr=DHCO3BDS(1) + u(1) * (DHCO3BDS(2) + u(1) * (DHCO3BDS(3) + u(1) * DHCO3BDS(4)))
  H2OVC : Fcn  Expr=u(1) + DH2ODS * u(2)
  H2OVC0 : Fcn  Expr=AH2OVC(1) + u(1) * AH2OVC(2)
  H2OVP : Fcn  Expr=H2OB - u(1)
  HCO3B : Fcn  Expr=u(2) + u(1) * u(3)
  HCO3B0 : Fcn  Expr=AHCO3B(1) + u(1) * (AHCO3B(2) + u(1) * (AHCO3B(3) + u(1) * AHCO3B(4)))
  HCO3P : Fcn  Expr=u(4) / (u(2) + u(1) * u(3))
  Hb sat0 : Fcn  Expr=u(1)*(150+u(1)*u(1))
  Hb sat1 : Fcn  Expr=u(1) /(23100+u(1))
  Mux{2..3,7..8,10} (5 alike) : Mux  Inputs=2
  Mux4 : Mux  Inputs=3
  Mux5 : Mux  Inputs=3
  Mux6 : Mux
  Mux9 : Mux  Inputs=3
  PCO2 : Product  OutDataType=sfix(16)  OutScaling=2^0  SaturateOnIntegerOverflow=on  RndMeth=Zero  InputSameDT=on  OutDataTypeStr=Inherit: Same as first input
  PCO2_37 : Product  OutDataType=sfix(16)  OutScaling=2^0  SaturateOnIntegerOverflow=on  RndMeth=Zero  InputSameDT=on  OutDataTypeStr=Inherit: Same as first input
  RATIO_PC_HC : Fcn  Expr=exp(LN10 * (u(1) - u(2))) / 0.0327
  RHCO3 : Fcn  Expr=u(1) + (2.805 + u(2) * (-0.2583) - u(1)) * u(3)
  RHCO30 : Fcn  Expr=3.658 + u(1) * (-0.3891)
  SCO2_B : Fcn  Expr=u(2) * 0.0362 + u(1) * 0.0327
  Sum : Sum  Inputs=-+  OutDataType=sfix(16)  OutScaling=2^0  SaturateOnIntegerOverflow=on  InputSameDT=on  OutDataTypeStr=Inherit: Same as first input
  Sum1 : Sum  Inputs=-+  OutDataType=sfix(16)  OutScaling=2^0  SaturateOnIntegerOverflow=on  InputSameDT=on  OutDataTypeStr=Inherit: Same as first input
  efectiveP : Fcn  Expr=u(1) * exp(LN10 * (BOHRF0 + BOHRF1 * u(2)));
  pH guess : simulink/Math Operations/Algebraic Constraint  SystemSampleTime=-1  z0=pH_guess
  pK : Fcn  Expr=-5.77601 + u(1) * (4.77908 + u(1) * (-0.634518 + u(1) * 0.0277776))
  C_CO2 : Outport  OutDataType=sfix(16)  OutScaling=2^0
  C_O2 : Outport  Port=2  OutDataType=sfix(16)  OutScaling=2^0
  wires:
  "C_O2 "/1 -> C_O2/1  "C_O2"
  Mux10/1 -> "C_O2 "/1
  PO2/1 -> Mux10/1, Mux2/1  "PO2"
  "C_CO2 "/1 -> C_CO2/1  "CCO2"
  SCO2_B/1 -> Mux9/2  "SCO2_B"
  Mux9/1 -> "C_CO2 "/1
  PCO2_37/1 -> Mux9/1, PCO2/2  "PCO2_37"
  HCO3B/1 -> Mux9/3, Mux6/4  "HCO3B"
  RATIO_PC_HC/1 -> PCO2_37/1  "RATIO_PC_HC"
  HCO3P/1 -> PCO2_37/2  "HCO3P"
  Hb sat1/1 -> Mux10/2, Sum/1  "HbSat"
  H2OVC/1 -> Mux8/2, Mux6/3, H2OVP/1  "H2OVC"
  Sum/1 -> Mux7/2, Mux4/1, Mux5/3  "DS"
  Constant2/1 -> Sum/2
  H2OVP/1 -> Mux8/1, Mux6/2  "H2OVP"
  Mux8/1 -> SCO2_B/1
  P_CO2/1 -> Sum1/2
  Sum1/1 -> pH guess/1
  Hb sat0/1 -> Hb sat1/1
  efectiveP/1 -> Hb sat0/1
  Mux2/1 -> efectiveP/1
  pH guess/1 -> Mux5/2, HCO3B0/1, DHCO3B/1, H2OVC0/1, RHCO30/1, Mux3/2, pK/1, Mux2/2  "pH"
  H2OVC0/1 -> Mux7/1  "H2OVC0"
  Mux7/1 -> H2OVC/1
  Mux4/1 -> HCO3B/1
  DHCO3B/1 -> Mux4/3
  HCO3B0/1 -> Mux4/2
  RHCO3/1 -> Mux6/1  "RHCO3"
  Mux6/1 -> HCO3P/1
  Constant3/1 -> PCO2/1  "Hb"
  pK/1 -> Mux3/1  "pK"
  RHCO30/1 -> Mux5/1
  Mux5/1 -> RHCO3/1
  Mux3/1 -> RATIO_PC_HC/1
  PCO2/1 -> Sum1/1  "PCO2"

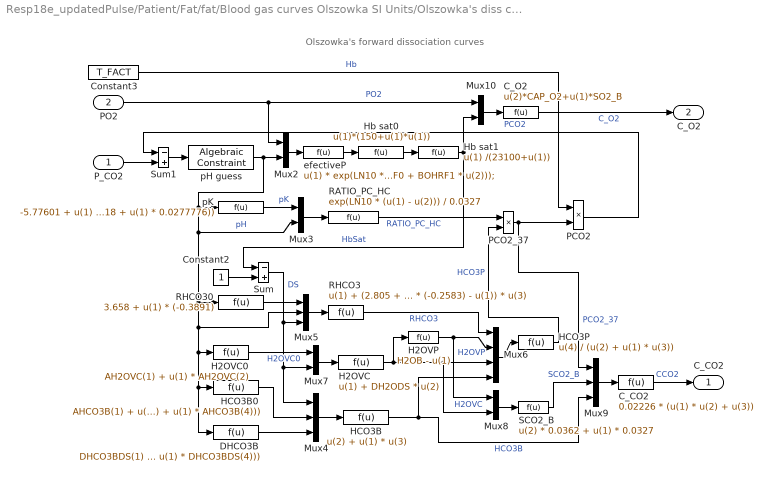
== system Resp18e_updatedPulse/Patient/Fat/fat/Blood gas curves Olszowka SI Units/Olszowka's diss curves ==
  note: Olszowka's forward dissociation curves
  P_CO2 : Inport  OutDataType=sfix(16)  OutScaling=2^0
  PO2 : Inport  Port=2  OutDataType=sfix(16)  OutScaling=2^0
  "C_CO2 " : Fcn  Expr=0.02226 * (u(1) * u(2) + u(3))
  "C_O2 " : Fcn  Expr=u(2)*CAP_O2+u(1)*SO2_B
  Constant2 : Constant  OutDataType=sfix(16)  OutScaling=2^0
  Constant3 : Constant  Value=T_FACT  OutDataType=sfix(16)  OutScaling=2^0
  DHCO3B : Fcn  Expr=DHCO3BDS(1) + u(1) * (DHCO3BDS(2) + u(1) * (DHCO3BDS(3) + u(1) * DHCO3BDS(4)))
  H2OVC : Fcn  Expr=u(1) + DH2ODS * u(2)
  H2OVC0 : Fcn  Expr=AH2OVC(1) + u(1) * AH2OVC(2)
  H2OVP : Fcn  Expr=H2OB - u(1)
  HCO3B : Fcn  Expr=u(2) + u(1) * u(3)
  HCO3B0 : Fcn  Expr=AHCO3B(1) + u(1) * (AHCO3B(2) + u(1) * (AHCO3B(3) + u(1) * AHCO3B(4)))
  HCO3P : Fcn  Expr=u(4) / (u(2) + u(1) * u(3))
  Hb sat0 : Fcn  Expr=u(1)*(150+u(1)*u(1))
  Hb sat1 : Fcn  Expr=u(1) /(23100+u(1))
  Mux{2..3,7..8,10} (5 alike) : Mux  Inputs=2
  Mux4 : Mux  Inputs=3
  Mux5 : Mux  Inputs=3
  Mux6 : Mux
  Mux9 : Mux  Inputs=3
  PCO2 : Product  OutDataType=sfix(16)  OutScaling=2^0  SaturateOnIntegerOverflow=on  RndMeth=Zero  InputSameDT=on  OutDataTypeStr=Inherit: Same as first input
  PCO2_37 : Product  OutDataType=sfix(16)  OutScaling=2^0  SaturateOnIntegerOverflow=on  RndMeth=Zero  InputSameDT=on  OutDataTypeStr=Inherit: Same as first input
  RATIO_PC_HC : Fcn  Expr=exp(LN10 * (u(1) - u(2))) / 0.0327
  RHCO3 : Fcn  Expr=u(1) + (2.805 + u(2) * (-0.2583) - u(1)) * u(3)
  RHCO30 : Fcn  Expr=3.658 + u(1) * (-0.3891)
  SCO2_B : Fcn  Expr=u(2) * 0.0362 + u(1) * 0.0327
  Sum : Sum  Inputs=-+  OutDataType=sfix(16)  OutScaling=2^0  SaturateOnIntegerOverflow=on  InputSameDT=on  OutDataTypeStr=Inherit: Same as first input
  Sum1 : Sum  Inputs=-+  OutDataType=sfix(16)  OutScaling=2^0  SaturateOnIntegerOverflow=on  InputSameDT=on  OutDataTypeStr=Inherit: Same as first input
  efectiveP : Fcn  Expr=u(1) * exp(LN10 * (BOHRF0 + BOHRF1 * u(2)));
  pH guess : simulink/Math Operations/Algebraic Constraint  SystemSampleTime=-1  z0=pH_guess
  pK : Fcn  Expr=-5.77601 + u(1) * (4.77908 + u(1) * (-0.634518 + u(1) * 0.0277776))
  C_CO2 : Outport  OutDataType=sfix(16)  OutScaling=2^0
  C_O2 : Outport  Port=2  OutDataType=sfix(16)  OutScaling=2^0
  wires:
  "C_O2 "/1 -> C_O2/1  "C_O2"
  Mux10/1 -> "C_O2 "/1
  PO2/1 -> Mux10/1, Mux2/1  "PO2"
  "C_CO2 "/1 -> C_CO2/1  "CCO2"
  SCO2_B/1 -> Mux9/2  "SCO2_B"
  Mux9/1 -> "C_CO2 "/1
  PCO2_37/1 -> Mux9/1, PCO2/2  "PCO2_37"
  HCO3B/1 -> Mux9/3, Mux6/4  "HCO3B"
  RATIO_PC_HC/1 -> PCO2_37/1  "RATIO_PC_HC"
  HCO3P/1 -> PCO2_37/2  "HCO3P"
  Hb sat1/1 -> Mux10/2, Sum/1  "HbSat"
  H2OVC/1 -> Mux8/2, Mux6/3, H2OVP/1  "H2OVC"
  Sum/1 -> Mux7/2, Mux4/1, Mux5/3  "DS"
  Constant2/1 -> Sum/2
  H2OVP/1 -> Mux8/1, Mux6/2  "H2OVP"
  Mux8/1 -> SCO2_B/1
  P_CO2/1 -> Sum1/2
  Sum1/1 -> pH guess/1
  Hb sat0/1 -> Hb sat1/1
  efectiveP/1 -> Hb sat0/1
  Mux2/1 -> efectiveP/1
  pH guess/1 -> Mux5/2, HCO3B0/1, DHCO3B/1, H2OVC0/1, RHCO30/1, Mux3/2, pK/1, Mux2/2  "pH"
  H2OVC0/1 -> Mux7/1  "H2OVC0"
  Mux7/1 -> H2OVC/1
  Mux4/1 -> HCO3B/1
  DHCO3B/1 -> Mux4/3
  HCO3B0/1 -> Mux4/2
  RHCO3/1 -> Mux6/1  "RHCO3"
  Mux6/1 -> HCO3P/1
  Constant3/1 -> PCO2/1  "Hb"
  pK/1 -> Mux3/1  "pK"
  RHCO30/1 -> Mux5/1
  Mux5/1 -> RHCO3/1
  Mux3/1 -> RATIO_PC_HC/1
  PCO2/1 -> Sum1/1  "PCO2"

== system Resp18e_updatedPulse/Patient/Heart/Heart/Blood gas curves Olszowka SI Units/Olszowka's diss curves ==
  note: Olszowka's forward dissociation curves
  P_CO2 : Inport  OutDataType=sfix(16)  OutScaling=2^0
  PO2 : Inport  Port=2  OutDataType=sfix(16)  OutScaling=2^0
  "C_CO2 " : Fcn  Expr=0.02226 * (u(1) * u(2) + u(3))
  "C_O2 " : Fcn  Expr=u(2)*CAP_O2+u(1)*SO2_B
  Constant2 : Constant  OutDataType=sfix(16)  OutScaling=2^0
  Constant3 : Constant  Value=T_FACT  OutDataType=sfix(16)  OutScaling=2^0
  DHCO3B : Fcn  Expr=DHCO3BDS(1) + u(1) * (DHCO3BDS(2) + u(1) * (DHCO3BDS(3) + u(1) * DHCO3BDS(4)))
  H2OVC : Fcn  Expr=u(1) + DH2ODS * u(2)
  H2OVC0 : Fcn  Expr=AH2OVC(1) + u(1) * AH2OVC(2)
  H2OVP : Fcn  Expr=H2OB - u(1)
  HCO3B : Fcn  Expr=u(2) + u(1) * u(3)
  HCO3B0 : Fcn  Expr=AHCO3B(1) + u(1) * (AHCO3B(2) + u(1) * (AHCO3B(3) + u(1) * AHCO3B(4)))
  HCO3P : Fcn  Expr=u(4) / (u(2) + u(1) * u(3))
  Hb sat0 : Fcn  Expr=u(1)*(150+u(1)*u(1))
  Hb sat1 : Fcn  Expr=u(1) /(23100+u(1))
  Mux{2..3,7..8,10} (5 alike) : Mux  Inputs=2
  Mux4 : Mux  Inputs=3
  Mux5 : Mux  Inputs=3
  Mux6 : Mux
  Mux9 : Mux  Inputs=3
  PCO2 : Product  OutDataType=sfix(16)  OutScaling=2^0  SaturateOnIntegerOverflow=on  RndMeth=Zero  InputSameDT=on  OutDataTypeStr=Inherit: Same as first input
  PCO2_37 : Product  OutDataType=sfix(16)  OutScaling=2^0  SaturateOnIntegerOverflow=on  RndMeth=Zero  InputSameDT=on  OutDataTypeStr=Inherit: Same as first input
  RATIO_PC_HC : Fcn  Expr=exp(LN10 * (u(1) - u(2))) / 0.0327
  RHCO3 : Fcn  Expr=u(1) + (2.805 + u(2) * (-0.2583) - u(1)) * u(3)
  RHCO30 : Fcn  Expr=3.658 + u(1) * (-0.3891)
  SCO2_B : Fcn  Expr=u(2) * 0.0362 + u(1) * 0.0327
  Sum : Sum  Inputs=-+  OutDataType=sfix(16)  OutScaling=2^0  SaturateOnIntegerOverflow=on  InputSameDT=on  OutDataTypeStr=Inherit: Same as first input
  Sum1 : Sum  Inputs=-+  OutDataType=sfix(16)  OutScaling=2^0  SaturateOnIntegerOverflow=on  InputSameDT=on  OutDataTypeStr=Inherit: Same as first input
  efectiveP : Fcn  Expr=u(1) * exp(LN10 * (BOHRF0 + BOHRF1 * u(2)));
  pH guess : simulink/Math Operations/Algebraic Constraint  SystemSampleTime=-1  z0=pH_guess
  pK : Fcn  Expr=-5.77601 + u(1) * (4.77908 + u(1) * (-0.634518 + u(1) * 0.0277776))
  C_CO2 : Outport  OutDataType=sfix(16)  OutScaling=2^0
  C_O2 : Outport  Port=2  OutDataType=sfix(16)  OutScaling=2^0
  wires:
  "C_O2 "/1 -> C_O2/1  "C_O2"
  Mux10/1 -> "C_O2 "/1
  PO2/1 -> Mux10/1, Mux2/1  "PO2"
  "C_CO2 "/1 -> C_CO2/1  "CCO2"
  SCO2_B/1 -> Mux9/2  "SCO2_B"
  Mux9/1 -> "C_CO2 "/1
  PCO2_37/1 -> Mux9/1, PCO2/2  "PCO2_37"
  HCO3B/1 -> Mux9/3, Mux6/4  "HCO3B"
  RATIO_PC_HC/1 -> PCO2_37/1  "RATIO_PC_HC"
  HCO3P/1 -> PCO2_37/2  "HCO3P"
  Hb sat1/1 -> Mux10/2, Sum/1  "HbSat"
  H2OVC/1 -> Mux8/2, Mux6/3, H2OVP/1  "H2OVC"
  Sum/1 -> Mux7/2, Mux4/1, Mux5/3  "DS"
  Constant2/1 -> Sum/2
  H2OVP/1 -> Mux8/1, Mux6/2  "H2OVP"
  Mux8/1 -> SCO2_B/1
  P_CO2/1 -> Sum1/2
  Sum1/1 -> pH guess/1
  Hb sat0/1 -> Hb sat1/1
  efectiveP/1 -> Hb sat0/1
  Mux2/1 -> efectiveP/1
  pH guess/1 -> Mux5/2, HCO3B0/1, DHCO3B/1, H2OVC0/1, RHCO30/1, Mux3/2, pK/1, Mux2/2  "pH"
  H2OVC0/1 -> Mux7/1  "H2OVC0"
  Mux7/1 -> H2OVC/1
  Mux4/1 -> HCO3B/1
  DHCO3B/1 -> Mux4/3
  HCO3B0/1 -> Mux4/2
  RHCO3/1 -> Mux6/1  "RHCO3"
  Mux6/1 -> HCO3P/1
  Constant3/1 -> PCO2/1  "Hb"
  pK/1 -> Mux3/1  "pK"
  RHCO30/1 -> Mux5/1
  Mux5/1 -> RHCO3/1
  Mux3/1 -> RATIO_PC_HC/1
  PCO2/1 -> Sum1/1  "PCO2"

== system Resp18e_updatedPulse/Patient/Kidneys/Kidneys/Blood gas curves Olszowka SI Units/Olszowka's diss curves ==
  note: Olszowka's forward dissociation curves
  P_CO2 : Inport  OutDataType=sfix(16)  OutScaling=2^0
  PO2 : Inport  Port=2  OutDataType=sfix(16)  OutScaling=2^0
  "C_CO2 " : Fcn  Expr=0.02226 * (u(1) * u(2) + u(3))
  "C_O2 " : Fcn  Expr=u(2)*CAP_O2+u(1)*SO2_B
  Constant2 : Constant  OutDataType=sfix(16)  OutScaling=2^0
  Constant3 : Constant  Value=T_FACT  OutDataType=sfix(16)  OutScaling=2^0
  DHCO3B : Fcn  Expr=DHCO3BDS(1) + u(1) * (DHCO3BDS(2) + u(1) * (DHCO3BDS(3) + u(1) * DHCO3BDS(4)))
  H2OVC : Fcn  Expr=u(1) + DH2ODS * u(2)
  H2OVC0 : Fcn  Expr=AH2OVC(1) + u(1) * AH2OVC(2)
  H2OVP : Fcn  Expr=H2OB - u(1)
  HCO3B : Fcn  Expr=u(2) + u(1) * u(3)
  HCO3B0 : Fcn  Expr=AHCO3B(1) + u(1) * (AHCO3B(2) + u(1) * (AHCO3B(3) + u(1) * AHCO3B(4)))
  HCO3P : Fcn  Expr=u(4) / (u(2) + u(1) * u(3))
  Hb sat0 : Fcn  Expr=u(1)*(150+u(1)*u(1))
  Hb sat1 : Fcn  Expr=u(1) /(23100+u(1))
  Mux{2..3,7..8,10} (5 alike) : Mux  Inputs=2
  Mux4 : Mux  Inputs=3
  Mux5 : Mux  Inputs=3
  Mux6 : Mux
  Mux9 : Mux  Inputs=3
  PCO2 : Product  OutDataType=sfix(16)  OutScaling=2^0  SaturateOnIntegerOverflow=on  RndMeth=Zero  InputSameDT=on  OutDataTypeStr=Inherit: Same as first input
  PCO2_37 : Product  OutDataType=sfix(16)  OutScaling=2^0  SaturateOnIntegerOverflow=on  RndMeth=Zero  InputSameDT=on  OutDataTypeStr=Inherit: Same as first input
  RATIO_PC_HC : Fcn  Expr=exp(LN10 * (u(1) - u(2))) / 0.0327
  RHCO3 : Fcn  Expr=u(1) + (2.805 + u(2) * (-0.2583) - u(1)) * u(3)
  RHCO30 : Fcn  Expr=3.658 + u(1) * (-0.3891)
  SCO2_B : Fcn  Expr=u(2) * 0.0362 + u(1) * 0.0327
  Sum : Sum  Inputs=-+  OutDataType=sfix(16)  OutScaling=2^0  SaturateOnIntegerOverflow=on  InputSameDT=on  OutDataTypeStr=Inherit: Same as first input
  Sum1 : Sum  Inputs=-+  OutDataType=sfix(16)  OutScaling=2^0  SaturateOnIntegerOverflow=on  InputSameDT=on  OutDataTypeStr=Inherit: Same as first input
  efectiveP : Fcn  Expr=u(1) * exp(LN10 * (BOHRF0 + BOHRF1 * u(2)));
  pH guess : simulink/Math Operations/Algebraic Constraint  SystemSampleTime=-1  z0=pH_guess
  pK : Fcn  Expr=-5.77601 + u(1) * (4.77908 + u(1) * (-0.634518 + u(1) * 0.0277776))
  C_CO2 : Outport  OutDataType=sfix(16)  OutScaling=2^0
  C_O2 : Outport  Port=2  OutDataType=sfix(16)  OutScaling=2^0
  wires:
  "C_O2 "/1 -> C_O2/1  "C_O2"
  Mux10/1 -> "C_O2 "/1
  PO2/1 -> Mux10/1, Mux2/1  "PO2"
  "C_CO2 "/1 -> C_CO2/1  "CCO2"
  SCO2_B/1 -> Mux9/2  "SCO2_B"
  Mux9/1 -> "C_CO2 "/1
  PCO2_37/1 -> Mux9/1, PCO2/2  "PCO2_37"
  HCO3B/1 -> Mux9/3, Mux6/4  "HCO3B"
  RATIO_PC_HC/1 -> PCO2_37/1  "RATIO_PC_HC"
  HCO3P/1 -> PCO2_37/2  "HCO3P"
  Hb sat1/1 -> Mux10/2, Sum/1  "HbSat"
  H2OVC/1 -> Mux8/2, Mux6/3, H2OVP/1  "H2OVC"
  Sum/1 -> Mux7/2, Mux4/1, Mux5/3  "DS"
  Constant2/1 -> Sum/2
  H2OVP/1 -> Mux8/1, Mux6/2  "H2OVP"
  Mux8/1 -> SCO2_B/1
  P_CO2/1 -> Sum1/2
  Sum1/1 -> pH guess/1
  Hb sat0/1 -> Hb sat1/1
  efectiveP/1 -> Hb sat0/1
  Mux2/1 -> efectiveP/1
  pH guess/1 -> Mux5/2, HCO3B0/1, DHCO3B/1, H2OVC0/1, RHCO30/1, Mux3/2, pK/1, Mux2/2  "pH"
  H2OVC0/1 -> Mux7/1  "H2OVC0"
  Mux7/1 -> H2OVC/1
  Mux4/1 -> HCO3B/1
  DHCO3B/1 -> Mux4/3
  HCO3B0/1 -> Mux4/2
  RHCO3/1 -> Mux6/1  "RHCO3"
  Mux6/1 -> HCO3P/1
  Constant3/1 -> PCO2/1  "Hb"
  pK/1 -> Mux3/1  "pK"
  RHCO30/1 -> Mux5/1
  Mux5/1 -> RHCO3/1
  Mux3/1 -> RATIO_PC_HC/1
  PCO2/1 -> Sum1/1  "PCO2"

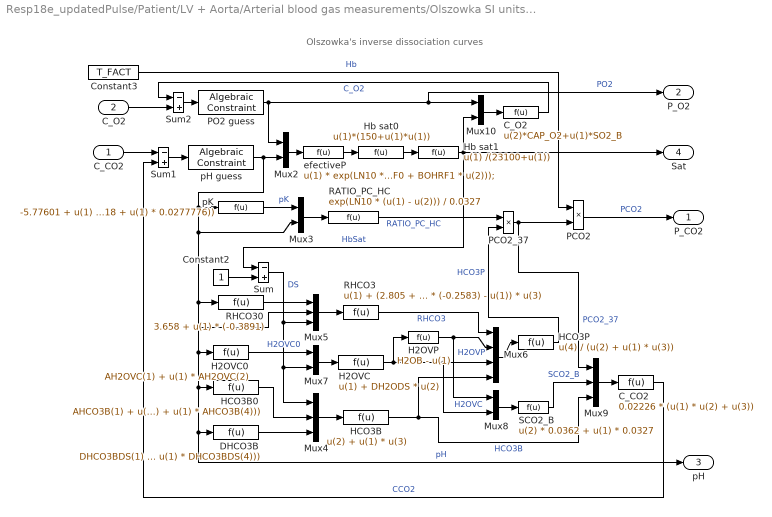
== system Resp18e_updatedPulse/Patient/LV + Aorta/Arterial blood gas measurements/Olszowka SI units/Olszowka's diss curves ==
  note: Olszowka's inverse dissociation curves
  C_CO2 : Inport  OutDataType=sfix(16)  OutScaling=2^0
  C_O2 : Inport  Port=2  OutDataType=sfix(16)  OutScaling=2^0
  "C_CO2 " : Fcn  Expr=0.02226 * (u(1) * u(2) + u(3))
  "C_O2 " : Fcn  Expr=u(2)*CAP_O2+u(1)*SO2_B
  Constant2 : Constant  OutDataType=sfix(16)  OutScaling=2^0
  Constant3 : Constant  Value=T_FACT  OutDataType=sfix(16)  OutScaling=2^0
  DHCO3B : Fcn  Expr=DHCO3BDS(1) + u(1) * (DHCO3BDS(2) + u(1) * (DHCO3BDS(3) + u(1) * DHCO3BDS(4)))
  H2OVC : Fcn  Expr=u(1) + DH2ODS * u(2)
  H2OVC0 : Fcn  Expr=AH2OVC(1) + u(1) * AH2OVC(2)
  H2OVP : Fcn  Expr=H2OB - u(1)
  HCO3B : Fcn  Expr=u(2) + u(1) * u(3)
  HCO3B0 : Fcn  Expr=AHCO3B(1) + u(1) * (AHCO3B(2) + u(1) * (AHCO3B(3) + u(1) * AHCO3B(4)))
  HCO3P : Fcn  Expr=u(4) / (u(2) + u(1) * u(3))
  Hb sat0 : Fcn  Expr=u(1)*(150+u(1)*u(1))
  Hb sat1 : Fcn  Expr=u(1) /(23100+u(1))
  Mux{2..3,7..8,10} (5 alike) : Mux  Inputs=2
  Mux4 : Mux  Inputs=3
  Mux5 : Mux  Inputs=3
  Mux6 : Mux
  Mux9 : Mux  Inputs=3
  PCO2 : Product  OutDataType=sfix(16)  OutScaling=2^0  SaturateOnIntegerOverflow=on  RndMeth=Zero  InputSameDT=on  OutDataTypeStr=Inherit: Same as first input
  PCO2_37 : Product  OutDataType=sfix(16)  OutScaling=2^0  SaturateOnIntegerOverflow=on  RndMeth=Zero  InputSameDT=on  OutDataTypeStr=Inherit: Same as first input
  PO2 guess : simulink/Math Operations/Algebraic Constraint  SystemSampleTime=-1  z0=P_O2_guess_inv
  RATIO_PC_HC : Fcn  Expr=exp(LN10 * (u(1) - u(2))) / 0.0327
  RHCO3 : Fcn  Expr=u(1) + (2.805 + u(2) * (-0.2583) - u(1)) * u(3)
  RHCO30 : Fcn  Expr=3.658 + u(1) * (-0.3891)
  SCO2_B : Fcn  Expr=u(2) * 0.0362 + u(1) * 0.0327
  Sum : Sum  Inputs=-+  OutDataType=sfix(16)  OutScaling=2^0  SaturateOnIntegerOverflow=on  InputSameDT=on  OutDataTypeStr=Inherit: Same as first input
  Sum1 : Sum  Inputs=-+  OutDataType=sfix(16)  OutScaling=2^0  SaturateOnIntegerOverflow=on  InputSameDT=on  OutDataTypeStr=Inherit: Same as first input
  Sum2 : Sum  Inputs=-+  OutDataType=sfix(16)  OutScaling=2^0  SaturateOnIntegerOverflow=on  InputSameDT=on  OutDataTypeStr=Inherit: Same as first input
  efectiveP : Fcn  Expr=u(1) * exp(LN10 * (BOHRF0 + BOHRF1 * u(2)));
  pH guess : simulink/Math Operations/Algebraic Constraint  SystemSampleTime=-1  z0=pH_guess_inv
  pK : Fcn  Expr=-5.77601 + u(1) * (4.77908 + u(1) * (-0.634518 + u(1) * 0.0277776))
  P_CO2 : Outport  OutDataType=sfix(16)  OutScaling=2^0
  P_O2 : Outport  Port=2  OutDataType=sfix(16)  OutScaling=2^0
  pH : Outport  Port=3  OutDataType=sfix(16)  OutScaling=2^0
  Sat : Outport  Port=4  OutDataType=sfix(16)  OutScaling=2^0
  wires:
  Mux3/1 -> RATIO_PC_HC/1
  Mux5/1 -> RHCO3/1
  RHCO30/1 -> Mux5/1
  pK/1 -> Mux3/1  "pK"
  Constant3/1 -> PCO2/1  "Hb"
  Mux6/1 -> HCO3P/1
  RHCO3/1 -> Mux6/1  "RHCO3"
  HCO3B0/1 -> Mux4/2
  DHCO3B/1 -> Mux4/3
  Mux4/1 -> HCO3B/1
  Mux7/1 -> H2OVC/1
  H2OVC0/1 -> Mux7/1  "H2OVC0"
  pH guess/1 -> Mux2/2, pK/1, Mux3/2, RHCO30/1, H2OVC0/1, HCO3B0/1, DHCO3B/1, pH/1, Mux5/2  "pH"
  Mux2/1 -> efectiveP/1
  efectiveP/1 -> Hb sat0/1
  Hb sat0/1 -> Hb sat1/1
  Sum1/1 -> pH guess/1
  Mux8/1 -> SCO2_B/1
  H2OVP/1 -> Mux6/2, Mux8/1  "H2OVP"
  Constant2/1 -> Sum/2
  Sum/1 -> Mux5/3, Mux4/1, Mux7/2  "DS"
  H2OVC/1 -> H2OVP/1, Mux6/3, Mux8/2  "H2OVC"
  Hb sat1/1 -> Sum/1, Mux10/2, Sat/1  "HbSat"
  HCO3P/1 -> PCO2_37/2  "HCO3P"
  RATIO_PC_HC/1 -> PCO2_37/1  "RATIO_PC_HC"
  HCO3B/1 -> Mux6/4, Mux9/3  "HCO3B"
  PCO2_37/1 -> PCO2/2, Mux9/1  "PCO2_37"
  Mux9/1 -> "C_CO2 "/1
  SCO2_B/1 -> Mux9/2  "SCO2_B"
  Mux10/1 -> "C_O2 "/1
  PCO2/1 -> P_CO2/1  "PCO2"
  Sum2/1 -> PO2 guess/1
  C_O2/1 -> Sum2/2
  PO2 guess/1 -> Mux2/1, Mux10/1, P_O2/1  "PO2"
  "C_O2 "/1 -> Sum2/1  "C_O2"
  "C_CO2 "/1 -> Sum1/2  "CCO2"
  C_CO2/1 -> Sum1/1
